simulink model "SOAR_integration_test"  (R2018b)
settings: Solver=VariableStepAuto  StartTime=0.0  StopTime=10.0  RelTol=1e-3
undefined symbols (not defined in the file): FSW_Lib, fswParams
libraries: sharedutil x3, dspmtrx3 x2, MEKF_lib x2, aerolibutil x2, actuators_lib x1, CDH_command_lib x1, Environment_lib x1, Mekf_joseph x1, actuator_processing_lib x1, allocation_lib x1, control_command_generation_lib x1, evironmentEstimation_lib x1
(part 1 of 2)
settings Model: Creator=devantormey  LastModifiedBy=devantormey

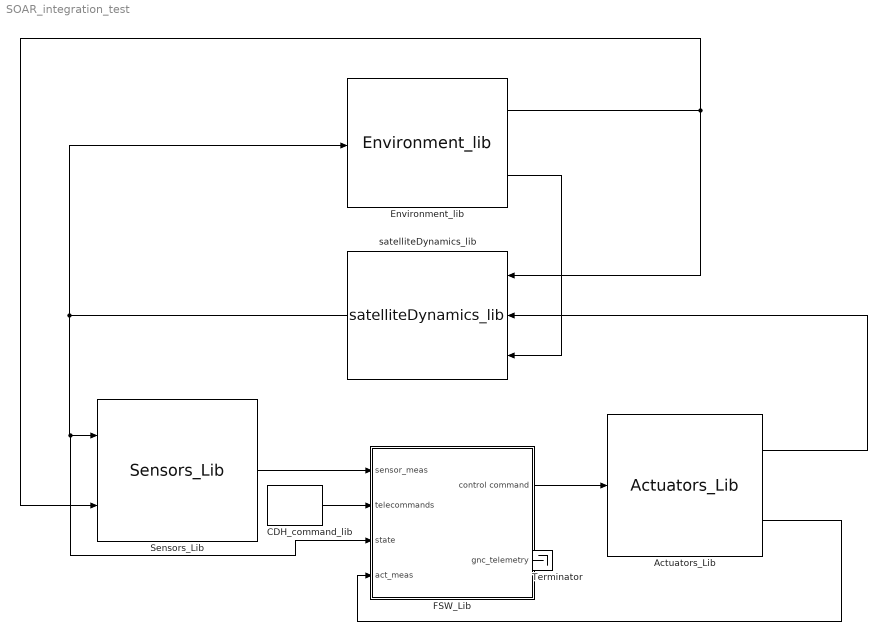
== system SOAR_integration_test ==
  Actuators_Lib : actuators_lib/Actuators_Lib  SystemSampleTime=-1
  CDH_command_lib : CDH_command_lib/CDH_command_lib  SystemSampleTime=-1
  Environment_lib : Environment_lib/Environment_lib  SystemSampleTime=-1
  FSW_Lib : Subsystem  AncestorBlock=FSW_Lib/FSW_Lib
  Sensors_Lib : Sensors_Lib/Sensors_Lib  SystemSampleTime=-1
  Terminator : Terminator
  satelliteDynamics_lib : satelliteDynamics_lib/satelliteDynamics_lib  SystemSampleTime=-1
  wires:
  Actuators_Lib/1 -> satelliteDynamics_lib/2
  FSW_Lib/2(gnc_telemetry) -> Terminator/1
  FSW_Lib/1(control command) -> Actuators_Lib/1
  Environment_lib/1 -> Sensors_Lib/2, satelliteDynamics_lib/1
  Environment_lib/2 -> satelliteDynamics_lib/3
  Sensors_Lib/1 -> FSW_Lib/1(sensor_meas)
  satelliteDynamics_lib/1 -> Environment_lib/1, FSW_Lib/3(state), Sensors_Lib/1
  Actuators_Lib/2 -> FSW_Lib/4(act_meas)
  CDH_command_lib/1 -> FSW_Lib/2(telecommands)

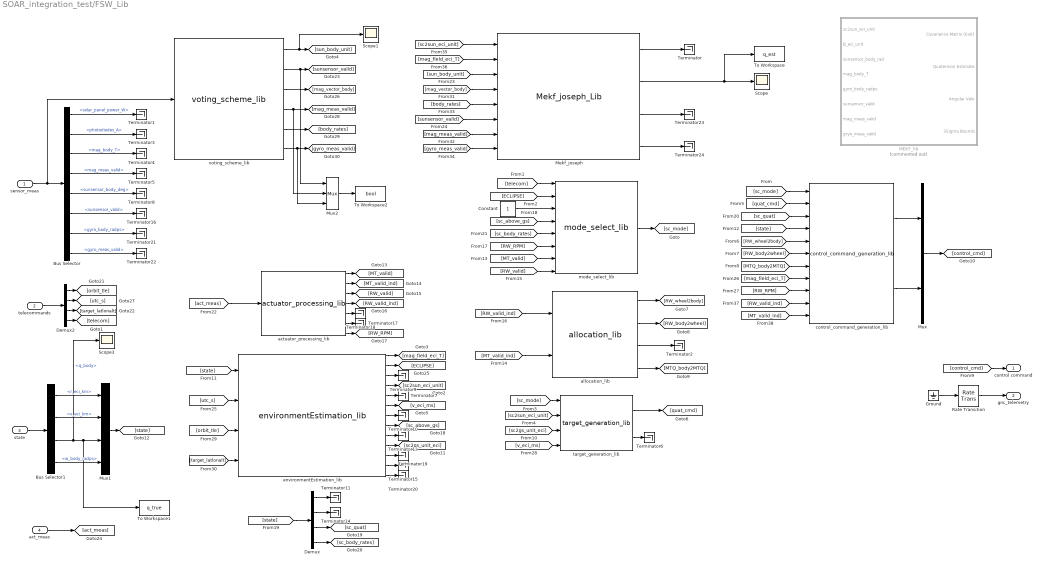
== system SOAR_integration_test/FSW_Lib ==
  sensor_meas : Inport
  telecommands : Inport  Port=2
  state : Inport  Port=3
  act_meas : Inport  Port=4
  Bus Selector : BusSelector  OutputSignals=solar_panel_power_W,photodiodes_A,mag_body_T,mag_meas_valid,sunsensor_body_deg,sunsensor_valid,gyro_body_radps,gyro_meas_valid
  Bus Selector1 : BusSelector  OutputSignals=r_eci_km,v_eci_km,q_body,w_body_radps
  Constant : Constant
  Demux : Demux  Outputs=[3 3 4 3]
  Demux2 : Demux  Outputs=[9 1 3 7]
  Ground : Ground
  MEKF_lib : Subsystem  Commented=on  AncestorBlock=MEKF_lib/MEKF_lib
  Mekf_joseph : Mekf_joseph/Mekf_joseph_Lib  SystemSampleTime=-1
      link override Data Store Memory: InitialValue=fswParams.estimation.ic.w_init
      link override "Subsystem Activated if: [Sun//Mag Sensor Invalid and Gyros are Valid] or [Gyro Invalid and Sun//Mag sensors Invalid]/TIME PROPAGATION of Q_EST, COVARIANCE": SourceBlock=Mekf_joseph/Mekf_joseph_Lib/Subsystem Activated if: [All Sensors Valid] or [Gyro Bad and Sun//Mag sensors Valid]/TIME PROPAGATION of Q_EST, COVARIANCE
  Mux : Mux  Inputs=[4 5]
  Mux1 : Mux  Inputs=[3;3;4;3]
  Mux2 : Mux  Inputs=3
  Rate Transition : RateTransition  OutPortSampleTime=fswParams.sample_time_s
  Scope : Scope
  Scope1 : Scope
  Scope3 : Scope
  Terminator{,1..11,13..24} (24 alike) : Terminator
  To Workspace : ToWorkspace  VariableName=q_est  SaveFormat=Timeseries  SampleTime=-1
  To Workspace1 : ToWorkspace  VariableName=q_true  SaveFormat=Timeseries  SampleTime=-1
  To Workspace2 : ToWorkspace  VariableName=bool  SaveFormat=Timeseries  SampleTime=-1
  actuator_processing_lib : actuator_processing_lib/actuator_processing_lib  SystemSampleTime=-1
  allocation_lib : allocation_lib/allocation_lib  SystemSampleTime=-1
  control_command_generation_lib : control_command_generation_lib/control_command_generation_lib  SystemSampleTime=-1
  environmentEstimation_lib : evironmentEstimation_lib/environmentEstimation_lib  SystemSampleTime=-1
      link override sgp4_lib_fsw/Gain: Gain=fswParams.constants.convert.KM2M
      link override sgp4_lib_fsw/Gain1: Gain=fswParams.constants.convert.KM2M
  mode_select_lib : mode_select_lib/mode_select_lib  SystemSampleTime=-1
  target_generation_lib : target_gen_lib/target_generation_lib  SystemSampleTime=-1
  voting_scheme_lib : voting_scheme_lib/voting_scheme_lib  SystemSampleTime=-1
  control command : Outport
  gnc_telemetry : Outport  Port=2
  wires:
  Rate Transition/1 -> gnc_telemetry/1
  target_generation_lib/1 -> [quat_cmd]
  [target_latlonalt] -> environmentEstimation_lib/4
  Demux2/3 -> [target_latlonalt]
  Demux2/1 -> [orbit_tle]
  [v_eci_ms] -> target_generation_lib/4
  [RW_RPM] -> control_command_generation_lib/9
  [mag_field_eci_T] -> control_command_generation_lib/8
  Demux2/2 -> [utc_s]
  Demux2/4 -> [telecom]
  environmentEstimation_lib/11 -> Terminator19/1
  environmentEstimation_lib/13 -> Terminator20/1
  environmentEstimation_lib/12 -> Terminator15/1
  Demux/2 -> Terminator14/1
  Demux/1 -> Terminator11/1
  Demux/4 -> [sc_body_rates]
  Demux/3 -> [sc_quat]
  [state] -> Demux/1
  actuator_processing_lib/7 -> [RW_RPM]
  actuator_processing_lib/6 -> Terminator17/1
  actuator_processing_lib/5 -> Terminator18/1
  actuator_processing_lib/4 -> [RW_valid_ind]
  actuator_processing_lib/3 -> [RW_valid]
  actuator_processing_lib/2 -> [MT_valid_ind]
  actuator_processing_lib/1 -> [MT_valid]
  act_meas/1 -> [act_meas]
  [state] -> control_command_generation_lib/4
  [state] -> environmentEstimation_lib/1
  [sc2gs_unit_eci] -> target_generation_lib/3
  [orbit_tle] -> environmentEstimation_lib/3
  [utc_s] -> environmentEstimation_lib/2
  environmentEstimation_lib/10 -> [sc2gs_unit_eci]
  environmentEstimation_lib/9 -> Terminator13/1
  environmentEstimation_lib/8 -> [sc_above_gs]
  environmentEstimation_lib/7 -> Terminator10/1
  environmentEstimation_lib/6 -> [v_eci_ms]
  environmentEstimation_lib/5 -> Terminator7/1
  environmentEstimation_lib/4 -> [sc2sun_eci_unit]
  environmentEstimation_lib/3 -> Terminator9/1
  environmentEstimation_lib/2 -> [ECLIPSE]
  environmentEstimation_lib/1 -> [mag_field_eci_T]
  Mux/1 -> [control_cmd]
  control_command_generation_lib/1 -> Mux/1
  control_command_generation_lib/2 -> Mux/2
  [MTQ_body2MTQ] -> control_command_generation_lib/7
  [RW_body2wheel] -> control_command_generation_lib/6
  allocation_lib/4 -> [MTQ_body2MTQ]
  allocation_lib/3 -> Terminator2/1
  [RW_wheel2body] -> control_command_generation_lib/5
  allocation_lib/2 -> [RW_body2wheel]
  allocation_lib/1 -> [RW_wheel2body]
  [sc_quat] -> control_command_generation_lib/3
  [MT_valid_ind] -> allocation_lib/2
  [RW_valid_ind] -> allocation_lib/1
  [quat_cmd] -> control_command_generation_lib/2
  target_generation_lib/2 -> Terminator6/1
  [sc2sun_eci_unit] -> target_generation_lib/2
  [sc_mode] -> target_generation_lib/1
  [RW_valid] -> mode_select_lib/8
  [MT_valid] -> mode_select_lib/7
  Constant/1 -> mode_select_lib/3
  [RW_RPM] -> mode_select_lib/6
  [sc_body_rates] -> mode_select_lib/5
  [sc_above_gs] -> mode_select_lib/4
  [ECLIPSE] -> mode_select_lib/2
  [telecom] -> mode_select_lib/1
  [sc_mode] -> control_command_generation_lib/1
  mode_select_lib/1 -> [sc_mode]
  [control_cmd] -> control command/1
  Ground/1 -> Rate Transition/1
  telecommands/1 -> Demux2/1
  sensor_meas/1 -> voting_scheme_lib/1, Bus Selector/1
  Bus Selector/1 -> Terminator1/1  "<solar_panel_power_W>"
  Bus Selector/2 -> Terminator3/1  "<photodiodes_A>"
  Bus Selector/3 -> Terminator4/1  "<mag_body_T>"
  Bus Selector/4 -> Terminator5/1  "<mag_meas_valid>"
  Bus Selector/5 -> Terminator8/1  "<sunsensor_body_deg>"
  Bus Selector/6 -> Terminator16/1  "<sunsensor_valid>"
  Bus Selector/7 -> Terminator21/1  "<gyro_body_radps>"
  Bus Selector/8 -> Terminator22/1  "<gyro_meas_valid>"
  voting_scheme_lib/3 -> [mag_vector_body]
  voting_scheme_lib/4 -> Mux2/2, [mag_meas_valid]
  voting_scheme_lib/5 -> [body_rates]
  voting_scheme_lib/6 -> Mux2/3, [gyro_meas_valid]
  [act_meas] -> actuator_processing_lib/1
  voting_scheme_lib/1 -> Scope1/1, [sun_body_unit]
  state/1 -> Bus Selector1/1
  Bus Selector1/1 -> Mux1/1  "<r_eci_km>"
  Bus Selector1/2 -> Mux1/2  "<v_eci_km>"
  Bus Selector1/3 -> To Workspace1/1, Mux1/3, Scope3/1  "<q_body>"
  Bus Selector1/4 -> Mux1/4  "<w_body_radps>"
  Mux1/1 -> [state]
  [sc2sun_eci_unit] -> Mekf_joseph/1
  [mag_field_eci_T] -> Mekf_joseph/2
  [body_rates] -> Mekf_joseph/5
  [mag_vector_body] -> Mekf_joseph/4
  [sunsensor_valid] -> Mekf_joseph/6
  [mag_meas_valid] -> Mekf_joseph/7
  [gyro_meas_valid] -> Mekf_joseph/8
  [sun_body_unit] -> Mekf_joseph/3
  Mekf_joseph/1 -> Terminator/1
  Mekf_joseph/2 -> Scope/1, To Workspace/1
  Mekf_joseph/3 -> Terminator23/1
  Mekf_joseph/4 -> Terminator24/1
  Mux2/1 -> To Workspace2/1
  voting_scheme_lib/2 -> Mux2/1, [sunsensor_valid]
  [RW_valid_ind] -> control_command_generation_lib/10
  [MT_valid_ind] -> control_command_generation_lib/11

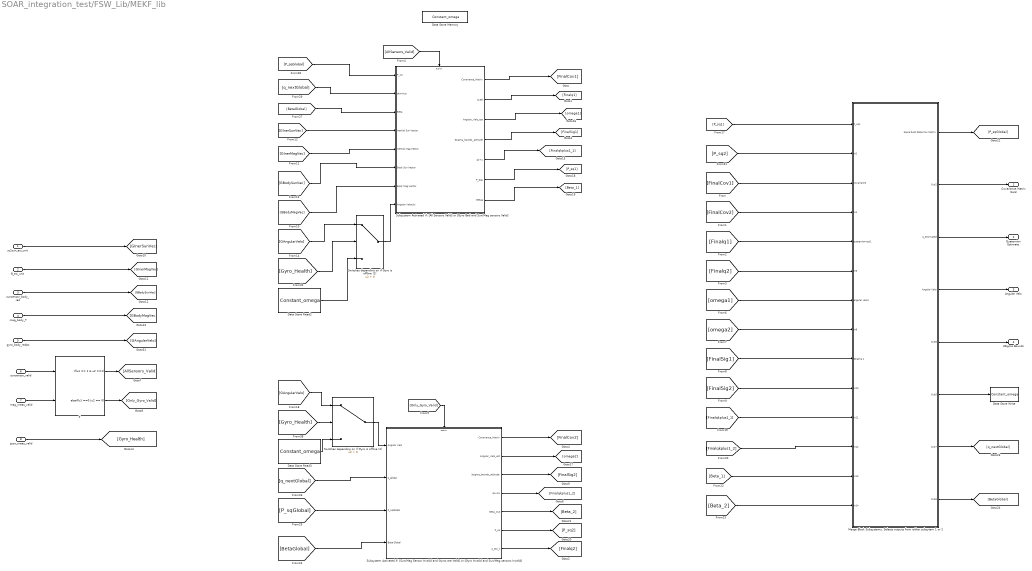
== system SOAR_integration_test/FSW_Lib/MEKF_lib ==
  sc2sun_eci_unit : Inport
  B_eci_unit : Inport  Port=2
  sunsensor_body_rad : Inport  Port=3
  mag_body_T : Inport  Port=4
  gyro_body_radps : Inport  Port=5
  sunsensor_valid : Inport  Port=6
  mag_meas_valid : Inport  Port=7
  gryo_meas_valid : Inport  Port=8
  Data Store Memory : DataStoreMemory  DataStoreName=Constant_omega  ReadBeforeWriteMsg=warning  WriteAfterWriteMsg=warning  WriteAfterReadMsg=warning  InitialValue=fswParams.estimation.ic.w_init  VectorParams1D=off  ShowAdditionalParam=off
  Data Store Read2 : DataStoreRead  DataStoreName=Constant_omega
  Data Store Read3 : DataStoreRead  DataStoreName=Constant_omega
  Data Store Write : DataStoreWrite  DataStoreName=Constant_omega
  If : If  NumInputs=2  IfExpression=u1 == 1 & u2 ==1  ElseIfExpressions=u1 ==0 |u2 == 0  ShowElse=off
  "Merge Block Subsystems, Selects outputs from either subsytem 1 or 2" : Subsystem
  Subsystem Activated if: [All Sensors Valid] or [Gyro Bad and Sun/Mag sensors Valid] : Subsystem  TreatAsAtomicUnit=on
  Subsystem Activated if: [Sun/Mag Sensor Invalid and Gyros are Valid] or [Gyro Invalid and Sun/Mag sensors Invalid] : Subsystem  TreatAsAtomicUnit=on
  Switches depending on if Gyro is offline (1) : Switch  Criteria=u2 > Threshold
  Switches depending on if Gyro is offline (2) : Switch  Criteria=u2 > Threshold
  Covariance Matrix (6x6) : Outport
  "Quaternion Estimate " : Outport  Port=2
  "Angular Velo " : Outport  Port=3
  "3Sigma Bounds " : Outport  Port=4
  wires:
  gyro_body_radps/1 -> [GAngularVelo]
  mag_body_T/1 -> [GBodyMagVec]
  B_eci_unit/1 -> [GInerMagVec]
  gryo_meas_valid/1 -> [Gyro_Health]
  mag_meas_valid/1 -> If/2
  sunsensor_valid/1 -> If/1
  sunsensor_body_rad/1 -> [GBodySunVec]
  sc2sun_eci_unit/1 -> [GInerSunVec]
  "Merge Block Subsystems, Selects outputs from either subsytem 1 or 2"/8(Out8) -> [BetaGlobal]
  "Merge Block Subsystems, Selects outputs from either subsytem 1 or 2"/7(Out7) -> [q_nextGlobal]
  "Merge Block Subsystems, Selects outputs from either subsytem 1 or 2"/5(Out6) -> "3Sigma Bounds "/1
  "Merge Block Subsystems, Selects outputs from either subsytem 1 or 2"/6(Out5) -> Data Store Write/1
  "Merge Block Subsystems, Selects outputs from either subsytem 1 or 2"/4(Angular Velo) -> "Angular Velo "/1
  "Merge Block Subsystems, Selects outputs from either subsytem 1 or 2"/3(q_estimated) -> "Quaternion Estimate "/1
  "Merge Block Subsystems, Selects outputs from either subsytem 1 or 2"/2(Out2) -> Covariance Matrix (6x6)/1
  "Merge Block Subsystems, Selects outputs from either subsytem 1 or 2"/1(Squre Root State Cov Matrix) -> [P_sqGlobal]
  [Beta_2] -> "Merge Block Subsystems, Selects outputs from either subsytem 1 or 2"/14(In14)
  [Beta_1] -> "Merge Block Subsystems, Selects outputs from either subsytem 1 or 2"/13(In13)
  [Finalqkplus1_2] -> "Merge Block Subsystems, Selects outputs from either subsytem 1 or 2"/12(In12)
  [Finalqkplus1_1] -> "Merge Block Subsystems, Selects outputs from either subsytem 1 or 2"/11(In11)
  [FinalSig2] -> "Merge Block Subsystems, Selects outputs from either subsytem 1 or 2"/10(In10)
  [FinalSig1] -> "Merge Block Subsystems, Selects outputs from either subsytem 1 or 2"/9(3sigma 1)
  [omega2] -> "Merge Block Subsystems, Selects outputs from either subsytem 1 or 2"/8(In8)
  [omega1] -> "Merge Block Subsystems, Selects outputs from either subsytem 1 or 2"/7(angular velo1)
  [Finalq2] -> "Merge Block Subsystems, Selects outputs from either subsytem 1 or 2"/6(In6)
  [Finalq1] -> "Merge Block Subsystems, Selects outputs from either subsytem 1 or 2"/5(quaternion est1)
  [FinalCov2] -> "Merge Block Subsystems, Selects outputs from either subsytem 1 or 2"/4(In4)
  [FinalCov1] -> "Merge Block Subsystems, Selects outputs from either subsytem 1 or 2"/3(covariance)
  [P_sq2] -> "Merge Block Subsystems, Selects outputs from either subsytem 1 or 2"/2(In2)
  [P_sq1] -> "Merge Block Subsystems, Selects outputs from either subsytem 1 or 2"/1(P_sq1)
  Switches depending on if Gyro is offline (2)/1 -> Subsystem Activated if: [Sun/Mag Sensor Invalid and Gyros are Valid] or [Gyro Invalid and Sun/Mag sensors Invalid]/1(Angular Velo)
  Data Store Read3/1 -> Switches depending on if Gyro is offline (2)/3
  [GAngularVelo] -> Switches depending on if Gyro is offline (2)/1
  [Gyro_Health] -> Switches depending on if Gyro is offline (2)/2
  Switches depending on if Gyro is offline (1)/1 -> Subsystem Activated if: [All Sensors Valid] or [Gyro Bad and Sun/Mag sensors Valid]/8(Angular Velocity)
  Data Store Read2/1 -> Switches depending on if Gyro is offline (1)/3
  [Gyro_Health] -> Switches depending on if Gyro is offline (1)/2
  [GAngularVelo] -> Switches depending on if Gyro is offline (1)/1
  If/2 -> [Only_Gyro_Valid]
  If/1 -> [AllSensors_Valid]
  [P_sqGlobal] -> Subsystem Activated if: [All Sensors Valid] or [Gyro Bad and Sun/Mag sensors Valid]/1(P_sq)
  [q_nextGlobal] -> Subsystem Activated if: [All Sensors Valid] or [Gyro Bad and Sun/Mag sensors Valid]/2(qkminus)
  Subsystem Activated if: [Sun/Mag Sensor Invalid and Gyros are Valid] or [Gyro Invalid and Sun/Mag sensors Invalid]/2(Angular_Velo_est) -> [omega2]
  Subsystem Activated if: [Sun/Mag Sensor Invalid and Gyros are Valid] or [Gyro Invalid and Sun/Mag sensors Invalid]/5(Beta_Out) -> [Beta_2]
  Subsystem Activated if: [Sun/Mag Sensor Invalid and Gyros are Valid] or [Gyro Invalid and Sun/Mag sensors Invalid]/6(P_sq) -> [P_sq2]
  Subsystem Activated if: [All Sensors Valid] or [Gyro Bad and Sun/Mag sensors Valid]/7(Betaa) -> [Beta_1]
  Subsystem Activated if: [All Sensors Valid] or [Gyro Bad and Sun/Mag sensors Valid]/6("P_Sqa ") -> [P_sq1]
  Subsystem Activated if: [All Sensors Valid] or [Gyro Bad and Sun/Mag sensors Valid]/3(Angular_Velo_est) -> [omega1]
  [BetaGlobal] -> Subsystem Activated if: [All Sensors Valid] or [Gyro Bad and Sun/Mag sensors Valid]/3(Beta)
  [BetaGlobal] -> Subsystem Activated if: [Sun/Mag Sensor Invalid and Gyros are Valid] or [Gyro Invalid and Sun/Mag sensors Invalid]/4(Beta Global)
  [P_sqGlobal] -> Subsystem Activated if: [Sun/Mag Sensor Invalid and Gyros are Valid] or [Gyro Invalid and Sun/Mag sensors Invalid]/3(P_sqGlobal)
  Subsystem Activated if: [All Sensors Valid] or [Gyro Bad and Sun/Mag sensors Valid]/5(qk+1) -> [Finalqkplus1_1]
  [q_nextGlobal] -> Subsystem Activated if: [Sun/Mag Sensor Invalid and Gyros are Valid] or [Gyro Invalid and Sun/Mag sensors Invalid]/2(q_global)
  Subsystem Activated if: [Sun/Mag Sensor Invalid and Gyros are Valid] or [Gyro Invalid and Sun/Mag sensors Invalid]/3(3sigma_bounds_attitude) -> [FinalSig2]
  [AllSensors_Valid] -> Subsystem Activated if: [All Sensors Valid] or [Gyro Bad and Sun/Mag sensors Valid]/Action
  Subsystem Activated if: [Sun/Mag Sensor Invalid and Gyros are Valid] or [Gyro Invalid and Sun/Mag sensors Invalid]/1(Covariance_Matrix) -> [FinalCov2]
  [GInerSunVec] -> Subsystem Activated if: [All Sensors Valid] or [Gyro Bad and Sun/Mag sensors Valid]/4(Inertial Sun Vector)
  Subsystem Activated if: [Sun/Mag Sensor Invalid and Gyros are Valid] or [Gyro Invalid and Sun/Mag sensors Invalid]/7(q_est_k) -> [Finalq2]
  Subsystem Activated if: [All Sensors Valid] or [Gyro Bad and Sun/Mag sensors Valid]/4(3sigma_bounds_attitude) -> [FinalSig1]
  [Only_Gyro_Valid] -> Subsystem Activated if: [Sun/Mag Sensor Invalid and Gyros are Valid] or [Gyro Invalid and Sun/Mag sensors Invalid]/Action
  Subsystem Activated if: [All Sensors Valid] or [Gyro Bad and Sun/Mag sensors Valid]/1(Covariance_Matrix) -> [FinalCov1]
  Subsystem Activated if: [All Sensors Valid] or [Gyro Bad and Sun/Mag sensors Valid]/2(q_est) -> [Finalq1]
  Subsystem Activated if: [Sun/Mag Sensor Invalid and Gyros are Valid] or [Gyro Invalid and Sun/Mag sensors Invalid]/4(qk+1a) -> [Finalqkplus1_2]
  [GBodyMagVec] -> Subsystem Activated if: [All Sensors Valid] or [Gyro Bad and Sun/Mag sensors Valid]/7(Body Mag Vector)
  [GInerMagVec] -> Subsystem Activated if: [All Sensors Valid] or [Gyro Bad and Sun/Mag sensors Valid]/5(Inertial Mag Vector)
  [GBodySunVec] -> Subsystem Activated if: [All Sensors Valid] or [Gyro Bad and Sun/Mag sensors Valid]/6(Body Sun Vector)

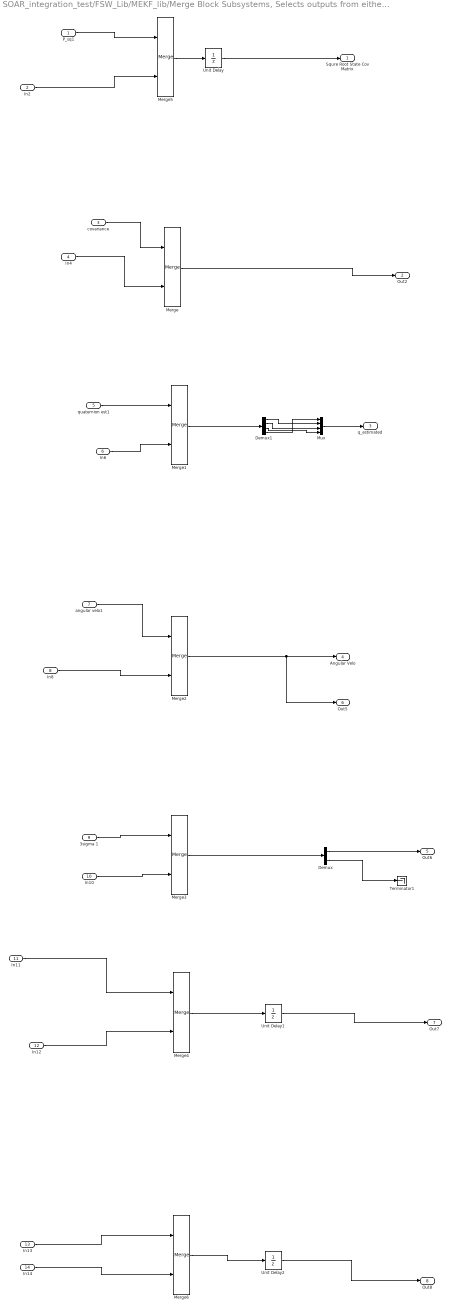
== system SOAR_integration_test/FSW_Lib/MEKF_lib/Merge Block Subsystems, Selects outputs from either subsytem 1 or 2 ==
  P_sq1 : Inport
  In2 : Inport  Port=2
  covariance : Inport  Port=3
  In4 : Inport  Port=4
  quaternion est1 : Inport  Port=5
  In6 : Inport  Port=6
  angular velo1 : Inport  Port=7
  In8 : Inport  Port=8
  3sigma 1 : Inport  Port=9
  In10 : Inport  Port=10
  In11 : Inport  Port=11
  In12 : Inport  Port=12
  In13 : Inport  Port=13
  In14 : Inport  Port=14
  Demux : Demux  Outputs=2
  Demux1 : Demux
  Merge{,1..6} (7 alike) : Merge
  Mux : Mux
  Terminator1 : Terminator
  Unit Delay : UnitDelay  InitialCondition=fswParams.estimation.ic.P_sq_init  SampleTime=-1
  Unit Delay1 : UnitDelay  InitialCondition=fswParams.estimation.ic.quat_est_init  SampleTime=-1
  Unit Delay2 : UnitDelay  InitialCondition=fswParams.estimation.ic.Beta_init  SampleTime=-1
  Squre Root State Cov Matrix : Outport
  Out2 : Outport  Port=2
  q_estimated : Outport  Port=3
  Angular Velo : Outport  Port=4
  Out6 : Outport  Port=5
  Out5 : Outport  Port=6
  Out7 : Outport  Port=7
  Out8 : Outport  Port=8
  wires:
  Mux/1 -> q_estimated/1
  Demux1/3 -> Mux/4
  Demux1/2 -> Mux/3
  Demux1/1 -> Mux/2
  Demux1/4 -> Mux/1
  Merge1/1 -> Demux1/1
  Unit Delay/1 -> Squre Root State Cov Matrix/1
  Unit Delay2/1 -> Out8/1
  P_sq1/1 -> Merge5/1
  In12/1 -> Merge4/2
  In8/1 -> Merge2/2
  In6/1 -> Merge1/2
  Merge/1 -> Out2/1
  In13/1 -> Merge6/1
  Demux/1 -> Out6/1
  In4/1 -> Merge/2
  Merge4/1 -> Unit Delay1/1
  covariance/1 -> Merge/1
  In2/1 -> Merge5/2
  In10/1 -> Merge3/2
  Merge5/1 -> Unit Delay/1
  In11/1 -> Merge4/1
  angular velo1/1 -> Merge2/1
  In14/1 -> Merge6/2
  quaternion est1/1 -> Merge1/1
  3sigma 1/1 -> Merge3/1
  Merge6/1 -> Unit Delay2/1
  Demux/2 -> Terminator1/1
  Unit Delay1/1 -> Out7/1
  Merge2/1 -> Angular Velo/1, Out5/1
  Merge3/1 -> Demux/1

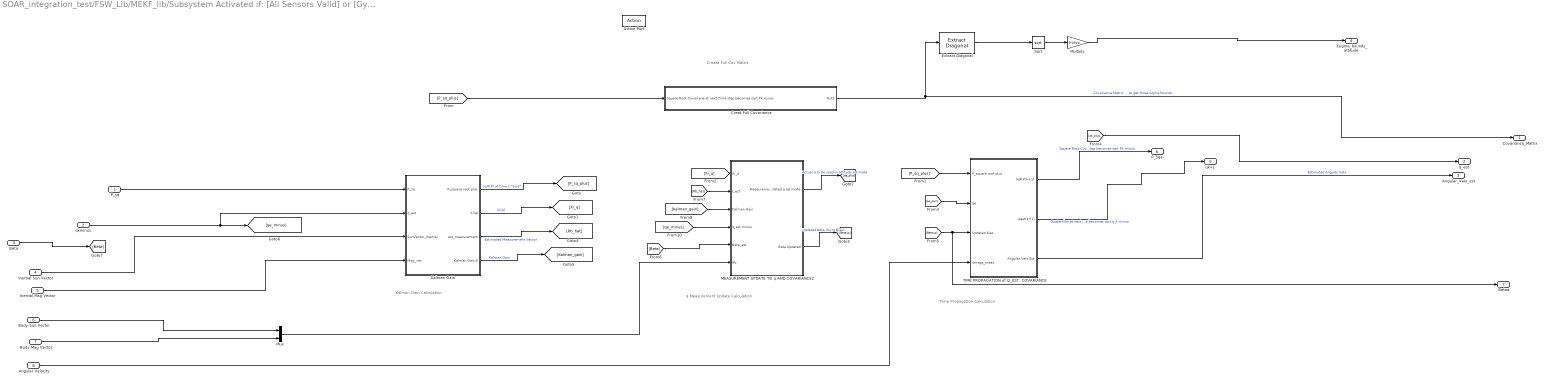
== system SOAR_integration_test/FSW_Lib/MEKF_lib/Subsystem Activated if: [All Sensors Valid] or [Gyro Bad and Sun//Mag sensors Valid] ==
  note: q Measurement Update Calculation
  note: Create Full Cov Matrix
  note: Time Propagation Calculation
  note: Kalman Gain Calculation
  P_sq : Inport
  qkminus : Inport  Port=2
  Beta : Inport  Port=3
  Inertial Sun Vector : Inport  Port=4
  Inertial Mag Vector : Inport  Port=5
  Body Sun Vector : Inport  Port=6
  Body Mag Vector : Inport  Port=7
  Angular Velocity : Inport  Port=8
  Action Port : ActionPort
  Creat Full Covariance : Subsystem  AncestorBlock=MEKF_LibraryR2018b/Multiplicative Extended Kalman Filter/Creat Full Covariance
  Extract Diagonal : dspmtrx3/Extract Diagonal
      settings: SourceProductName=DSP System Toolbox  SourceProductBaseCode=DS
  Kalman Gain : Subsystem  AncestorBlock=MEKF_LibraryR2018b/Multiplicative Extended Kalman Filter/Kalman Gain
  MEASUREMENT UPDATE TO q AND COVARIANCE2 : Subsystem  AncestorBlock=MEKF_LibraryR2018b/Multiplicative Extended Kalman Filter/MEASUREMENT UPDATE TO q AND COVARIANCE2
  Multiply : Gain  Gain=3*180/pi
  Mux : Mux  Inputs=2
  Sqrt : Sqrt  SaturateOnIntegerOverflow=on
  "TIME PROPAGATION of Q_EST, COVARIANCE" : Subsystem  AncestorBlock=MEKF_Library/Multiplicative Extended Kalman Filter/TIME PROPAGATION of Q_EST, COVARIANCE
  Covariance_Matrix : Outport
  q_est : Outport  Port=2
  Angular_Velo_est : Outport  Port=3
  3sigma_bounds_attitude : Outport  Port=4
  qk+1 : Outport  Port=5
  "P_Sqa " : Outport  Port=6
  Betaa : Outport  Port=7
  wires:
  Beta/1 -> [Beta]
  Multiply/1 -> 3sigma_bounds_attitude/1
  Mux/1 -> MEASUREMENT UPDATE TO q AND COVARIANCE2/6(Rb)
  Body Mag Vector/1 -> Mux/2
  Body Sun Vector/1 -> Mux/1
  Inertial Mag Vector/1 -> Kalman Gain/4("Mag_vec ")
  [Kalman_gain] -> MEASUREMENT UPDATE TO q AND COVARIANCE2/3(Kalman Gain)
  [Xi_q] -> MEASUREMENT UPDATE TO q AND COVARIANCE2/1(Xi_q)
  Kalman Gain/3(est_measurement) -> [Rb_hat]  "Estimated Measurement Vector"
  [P_sq_plus] -> "TIME PROPAGATION of Q_EST, COVARIANCE"/1(P_square root plus)
  MEASUREMENT UPDATE TO q AND COVARIANCE2/1(Measurement updated q estimate) -> [qe_plus]  "Actual q to be used in attitude estimate"
  [Beta] -> MEASUREMENT UPDATE TO q AND COVARIANCE2/5(Beta_est)
  [Betaup] -> "TIME PROPAGATION of Q_EST, COVARIANCE"/3(Updated bias), Betaa/1
  [P_sq_plus] -> Creat Full Covariance/1(Square Root Covariane at next Time step becomes sqrt Pk minus)
  Sqrt/1 -> Multiply/1
  Kalman Gain/2(Xi(q)) -> [Xi_q]  "Xi(q)"
  [qe_minus] -> MEASUREMENT UPDATE TO q AND COVARIANCE2/4(q_est minus)
  Kalman Gain/4(Kalman Gain K) -> [Kalman_gain]  "Kalman Gain"
  Kalman Gain/1(P_square root plus) -> [P_sq_plus]  "sqrt(P) at time k *plus*"
  "TIME PROPAGATION of Q_EST, COVARIANCE"/1(SqR P(k+1)) -> "P_Sqa "/1  "Square Root Covariane at next Time step becomes sqrt Pk minus"
  [Rb_hat] -> MEASUREMENT UPDATE TO q AND COVARIANCE2/2(r_est)
  MEASUREMENT UPDATE TO q AND COVARIANCE2/2(Beta Updated) -> [Betaup]  "Updated Beta (Gyro Bias)"
  [qe_plus] -> "TIME PROPAGATION of Q_EST, COVARIANCE"/2(qe)
  P_sq/1 -> Kalman Gain/1(P_sq)
  Angular Velocity/1 -> "TIME PROPAGATION of Q_EST, COVARIANCE"/4(omega_meas)
  Extract Diagonal/1 -> Sqrt/1
  qkminus/1 -> [qe_minus], Kalman Gain/2(q_est)
  Creat Full Covariance/1(Out1) -> Extract Diagonal/1, Covariance_Matrix/1  "Covariance Matrix from which to get three sigma bounds"
  "TIME PROPAGATION of Q_EST, COVARIANCE"/3(Angular Velo Est) -> Angular_Velo_est/1  "Estimated Angular Velo"
  "TIME PROPAGATION of Q_EST, COVARIANCE"/2(qest(k+1)) -> qk+1/1  "Quaternion at next Time step becomes sqrt q_k minus"
  [qe_plus] -> q_est/1
  Inertial Sun Vector/1 -> Kalman Gain/3(SunVector_Inertial)

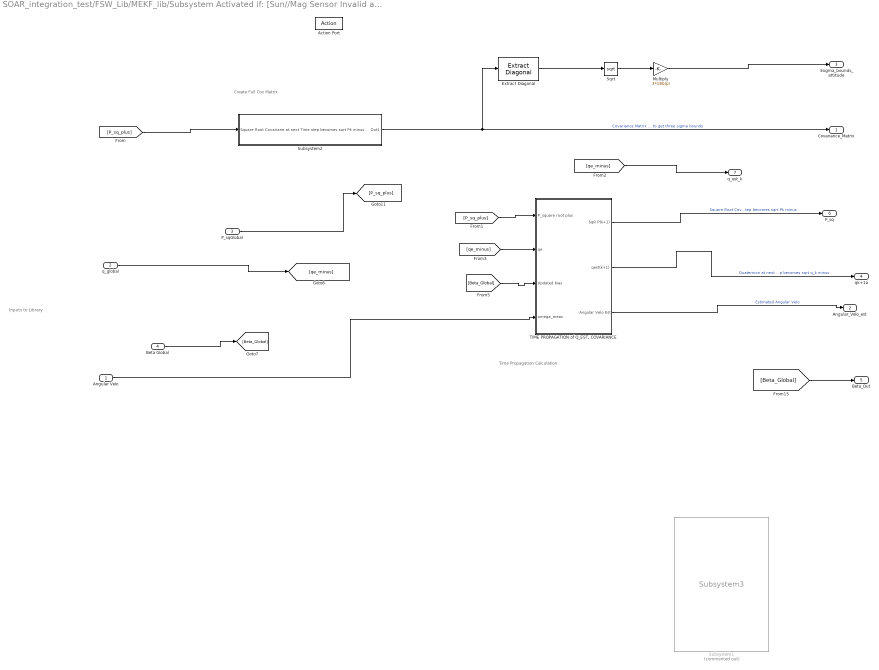
== system SOAR_integration_test/FSW_Lib/MEKF_lib/Subsystem Activated if: [Sun//Mag Sensor Invalid and Gyros are Valid] or [Gyro Invalid and Sun//Mag sensors Invalid] ==
  note: Time Propagation Calculation
  note: Inputs to Library
  note: Create Full Cov Matrix
  Angular Velo : Inport
  q_global : Inport  Port=2
  P_sqGlobal : Inport  Port=3
  Beta Global : Inport  Port=4
  Action Port : ActionPort
  Extract Diagonal : dspmtrx3/Extract Diagonal
      settings: SourceProductName=DSP System Toolbox  SourceProductBaseCode=DS
  Multiply : Gain  Gain=3*180/pi
  Sqrt : Sqrt  SaturateOnIntegerOverflow=on
  Subsystem1 : MEKF_lib/MEKF with Validity Check/Subsystem Activated if: [Sun//Mag Sensor Invalid and Gyros are Valid] or [Gyro Invalid and Sun//Mag sensors Invalid]/Subsystem3  Commented=on  SystemSampleTime=-1  SSRTWFcnClass=[]
  Subsystem2 : Subsystem
  "TIME PROPAGATION of Q_EST, COVARIANCE" : Subsystem  AncestorBlock=|
      | MEKF_SensorCheck_Lib2018/MEKF with Validity Check/Subsystem Activated if: [All Sensors Valid]
      | or
      | [Gyro Bad and Sun//Mag sensors Valid]/TIME PROPAGATION of Q_EST, COVARIANCE
  Covariance_Matrix : Outport
  Angular_Velo_est : Outport  Port=2
  3sigma_bounds_attitude : Outport  Port=3
  qk+1a : Outport  Port=4
  Beta_Out : Outport  Port=5
  P_sq : Outport  Port=6
  q_est_k : Outport  Port=7
  wires:
  [qe_minus] -> q_est_k/1
  [Beta_Global] -> Beta_Out/1
  Beta Global/1 -> [Beta_Global]
  "TIME PROPAGATION of Q_EST, COVARIANCE"/1(SqR P(k+1)) -> P_sq/1  "Square Root Covariane at next Time step becomes sqrt Pk minus"
  Multiply/1 -> 3sigma_bounds_attitude/1
  Angular Velo/1 -> "TIME PROPAGATION of Q_EST, COVARIANCE"/4(omega_meas)
  q_global/1 -> [qe_minus]
  Extract Diagonal/1 -> Sqrt/1
  [Beta_Global] -> "TIME PROPAGATION of Q_EST, COVARIANCE"/3(Updated bias)
  [P_sq_plus] -> "TIME PROPAGATION of Q_EST, COVARIANCE"/1(P_square root plus)
  [P_sq_plus] -> Subsystem2/1(Square Root Covariane at next Time step becomes sqrt Pk minus)
  "TIME PROPAGATION of Q_EST, COVARIANCE"/3(Angular Velo Est) -> Angular_Velo_est/1  "Estimated Angular Velo"
  Subsystem2/1(Out1) -> Extract Diagonal/1, Covariance_Matrix/1  "Covariance Matrix from which to get three sigma bounds"
  Sqrt/1 -> Multiply/1
  "TIME PROPAGATION of Q_EST, COVARIANCE"/2(qest(k+1)) -> qk+1a/1  "Quaternion at next Time step becomes sqrt q_k minus"
  [qe_minus] -> "TIME PROPAGATION of Q_EST, COVARIANCE"/2(qe)
  P_sqGlobal/1 -> [P_sq_plus]

== system SOAR_integration_test/FSW_Lib/MEKF_lib/Subsystem Activated if: [All Sensors Valid] or [Gyro Bad and Sun//Mag sensors Valid]/Creat Full Covariance ==
  Square Root Covariane at next Time step becomes sqrt Pk minus : Inport
  Matrix Multiply : Product  Multiplication=Matrix(*)
  Transpose : Math  Operator=transpose  SaturateOnIntegerOverflow=on
  Out1 : Outport
  wires:
  Matrix Multiply/1 -> Out1/1
  Transpose/1 -> Matrix Multiply/2
  Square Root Covariane at next Time step becomes sqrt Pk minus/1 -> Matrix Multiply/1, Transpose/1

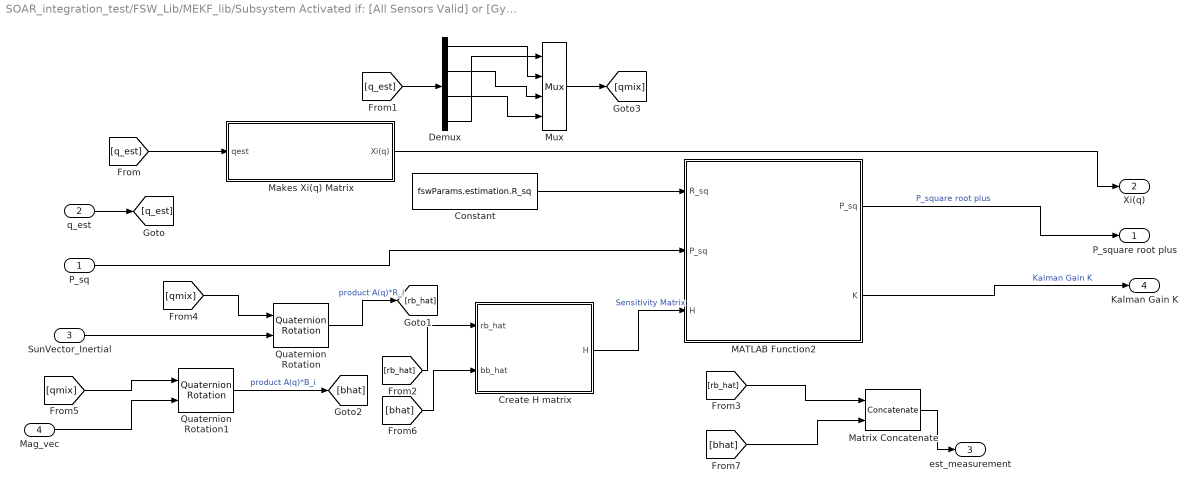
== system SOAR_integration_test/FSW_Lib/MEKF_lib/Subsystem Activated if: [All Sensors Valid] or [Gyro Bad and Sun//Mag sensors Valid]/Kalman Gain ==
  P_sq : Inport
  q_est : Inport  Port=2
  SunVector_Inertial : Inport  Port=3
  "Mag_vec " : Inport  Port=4
  Constant : Constant  Value=fswParams.estimation.R_sq  VectorParams1D=off
  Create H matrix : Subsystem
  Demux : Demux
  MATLAB Function2 : MATLAB Function  TreatAsAtomicUnit=on
  Makes Xi(q) Matrix : Subsystem
  Matrix Concatenate : Concatenate  Mode=Multidimensional array
  Mux : Mux
  Quaternion Rotation : aerolibutil/Quaternion Rotation
  Quaternion Rotation1 : aerolibutil/Quaternion Rotation
  P_square root plus : Outport
  Xi(q) : Outport  Port=2
  est_measurement : Outport  Port=3
  Kalman Gain K : Outport  Port=4
  wires:
  Matrix Concatenate/1 -> est_measurement/1
  [bhat] -> Matrix Concatenate/2
  [rb_hat] -> Matrix Concatenate/1
  [bhat] -> Create H matrix/2(bb_hat)
  [qmix] -> Quaternion Rotation/1
  [qmix] -> Quaternion Rotation1/1
  Mux/1 -> [qmix]
  Quaternion Rotation1/1 -> [bhat]  "product A(q)*B_i"
  "Mag_vec "/1 -> Quaternion Rotation1/2
  [rb_hat] -> Create H matrix/1(rb_hat)
  Quaternion Rotation/1 -> [rb_hat]  "product A(q)*R_i"
  [q_est] -> Makes Xi(q) Matrix/1(qest)
  [q_est] -> Demux/1
  q_est/1 -> [q_est]
  Makes Xi(q) Matrix/1(Xi(q)) -> Xi(q)/1
  Demux/4 -> Mux/1
  Demux/3 -> Mux/4
  Demux/2 -> Mux/3
  Demux/1 -> Mux/2
  MATLAB Function2/1(P_sq) -> P_square root plus/1  "P_square root plus"
  Constant/1 -> MATLAB Function2/1(R_sq)
  SunVector_Inertial/1 -> Quaternion Rotation/2
  MATLAB Function2/2(K) -> Kalman Gain K/1  "Kalman Gain K"
  P_sq/1 -> MATLAB Function2/2("P_sq ")
  Create H matrix/1(H) -> MATLAB Function2/3(H)  "Sensitivity Matrix"

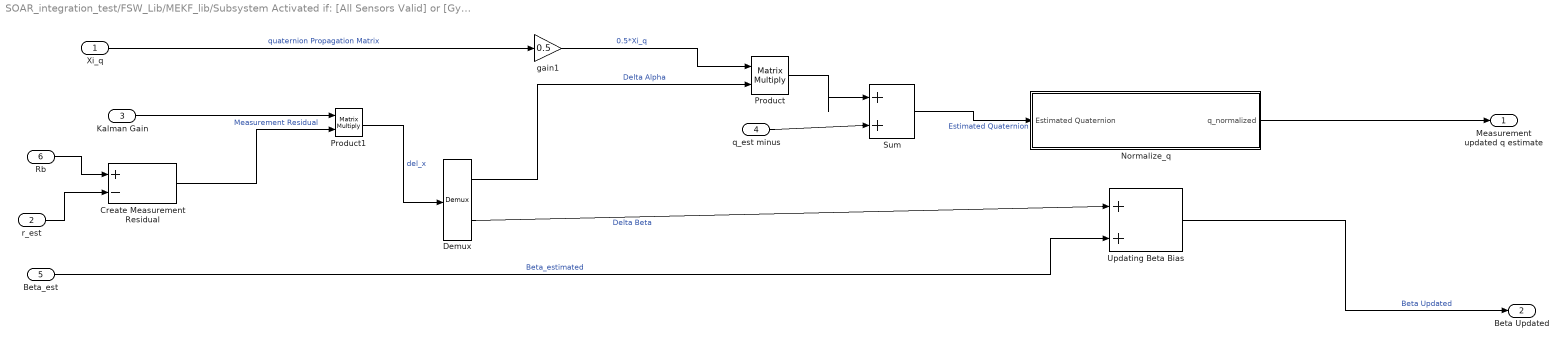
== system SOAR_integration_test/FSW_Lib/MEKF_lib/Subsystem Activated if: [All Sensors Valid] or [Gyro Bad and Sun//Mag sensors Valid]/MEASUREMENT UPDATE TO q AND COVARIANCE2 ==
  Xi_q : Inport
  r_est : Inport  Port=2
  Kalman Gain : Inport  Port=3
  q_est minus : Inport  Port=4
  Beta_est : Inport  Port=5
  Rb : Inport  Port=6
  Create Measurement Residual : Sum  Inputs=+-
  Demux : Demux  Outputs=2
  Normalize_q : Subsystem
  Product : Product  Inputs=**  Multiplication=Matrix(*)
  Product1 : Product  Multiplication=Matrix(*)
  Sum : Sum  Inputs=|++
  "Updating Beta Bias " : Sum  Inputs=|++
  gain1 : Gain  Gain=0.5
  Measurement updated q estimate : Outport
  Beta Updated : Outport  Port=2
  wires:
  Normalize_q/1(q_normalized) -> Measurement updated q estimate/1
  Sum/1 -> Normalize_q/1(Estimated Quaternion)  "Estimated Quaternion"
  Xi_q/1 -> gain1/1  "quaternion Propagation Matrix"
  Rb/1 -> Create Measurement Residual/1
  Kalman Gain/1 -> Product1/1
  q_est minus/1 -> Sum/2
  Beta_est/1 -> "Updating Beta Bias "/2  "Beta_estimated"
  "Updating Beta Bias "/1 -> Beta Updated/1  "Beta Updated"
  Create Measurement Residual/1 -> Product1/2  "Measurement Residual"
  r_est/1 -> Create Measurement Residual/2
  Product1/1 -> Demux/1  "del_x"
  Product/1 -> Sum/1
  Demux/2 -> "Updating Beta Bias "/1  "Delta Beta"
  gain1/1 -> Product/1  "0.5*Xi_q"
  Demux/1 -> Product/2  "Delta Alpha"

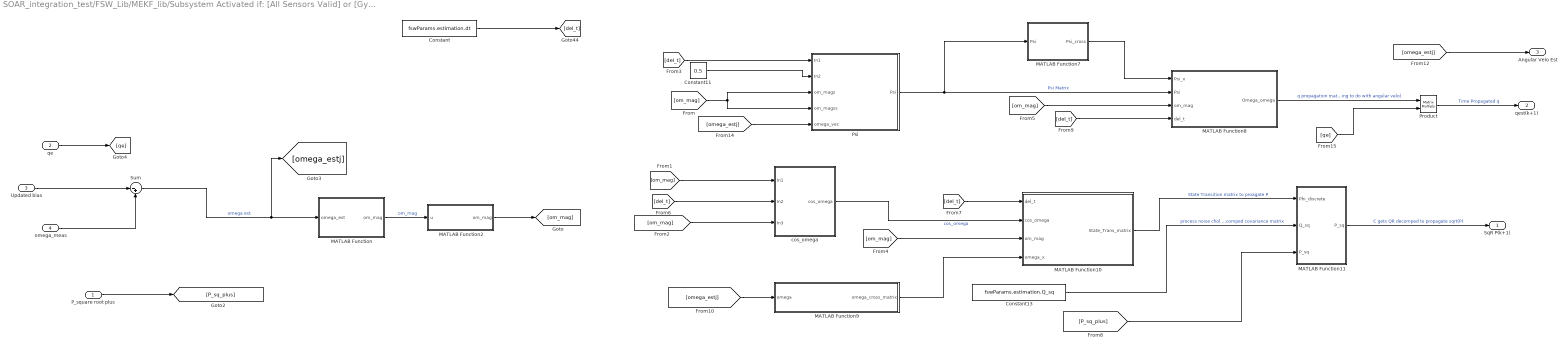
== system SOAR_integration_test/FSW_Lib/MEKF_lib/Subsystem Activated if: [All Sensors Valid] or [Gyro Bad and Sun//Mag sensors Valid]/TIME PROPAGATION of Q_EST, COVARIANCE ==
  P_square root plus : Inport
  qe : Inport  Port=2
  Updated bias : Inport  Port=3
  omega_meas : Inport  Port=4
  Constant : Constant  Value=fswParams.estimation.dt
  Constant11 : Constant  Value=0.5
  Constant13 : Constant  Value=fswParams.estimation.Q_sq  VectorParams1D=off
  MATLAB Function : MATLAB Function  TreatAsAtomicUnit=on
  MATLAB Function10 : MATLAB Function  TreatAsAtomicUnit=on
  MATLAB Function11 : MATLAB Function  TreatAsAtomicUnit=on
  MATLAB Function2 : MATLAB Function  TreatAsAtomicUnit=on
  MATLAB Function7 : MATLAB Function  TreatAsAtomicUnit=on
  MATLAB Function8 : MATLAB Function  TreatAsAtomicUnit=on
  MATLAB Function9 : MATLAB Function  TreatAsAtomicUnit=on
  Product : Product  Multiplication=Matrix(*)
  Psi : Subsystem
  Sum : Sum  Inputs=|-+
  cos_omega : Subsystem
  SqR P(k+1) : Outport
  qest(k+1) : Outport  Port=2
  Angular Velo Est : Outport  Port=3
  wires:
  MATLAB Function2/1(om_mag) -> [om_mag]
  [del_t] -> cos_omega/2(In2)
  Sum/1 -> MATLAB Function/1(omega_est), [omega_estj]  "omega est"
  [om_mag] -> Psi/4(om_magss), Psi/3(om_mags)
  [omega_estj] -> Psi/5(omega_vec)
  Constant11/1 -> Psi/2(In2)
  [del_t] -> Psi/1(In1)
  Psi/1(Psi) -> MATLAB Function7/1(Psi), MATLAB Function8/2(Psi)  "Psi Matrix"
  cos_omega/1(cos_omega) -> MATLAB Function10/2(cos_omega)  "cos_omega"
  [om_mag] -> cos_omega/3(In3)
  [om_mag] -> cos_omega/1(In1)
  [qe] -> Product/2
  [omega_estj] -> MATLAB Function9/1(omega)
  [om_mag] -> MATLAB Function8/3(om_mag)
  MATLAB Function/1(om_mag) -> MATLAB Function2/1(u)  "om_mag"
  Constant13/1 -> MATLAB Function11/2(Q_sq)  "process noise chol decomped covariance matrix"
  Product/1 -> qest(k+1)/1  "Time Propagated q"
  MATLAB Function10/1(State_Trans_matrix) -> MATLAB Function11/1(Phi_discrete)  "State Transition matrix to proagate P"
  MATLAB Function9/1(omega_cross_matrix) -> MATLAB Function10/4(omega_x)
  MATLAB Function8/1(Omega_omega) -> Product/1  "q propagation matrix (nothing to do with angular velo)"
  MATLAB Function11/1(P_sq) -> SqR P(k+1)/1  "C gets QR decomped to propagate sqrt(P)"
  MATLAB Function7/1(Psi_cross) -> MATLAB Function8/1(Psi_x)
  [del_t] -> MATLAB Function8/4(del_t)
  qe/1 -> [qe]
  Updated bias/1 -> Sum/1
  omega_meas/1 -> Sum/2
  P_square root plus/1 -> [P_sq_plus]
  [omega_estj] -> Angular Velo Est/1
  Constant/1 -> [del_t]
  [del_t] -> MATLAB Function10/1(del_t)
  [om_mag] -> MATLAB Function10/3(om_mag)
  [P_sq_plus] -> MATLAB Function11/3("P_sq ")

== system SOAR_integration_test/FSW_Lib/MEKF_lib/Subsystem Activated if: [Sun//Mag Sensor Invalid and Gyros are Valid] or [Gyro Invalid and Sun//Mag sensors Invalid]/Subsystem2 ==
  Square Root Covariane at next Time step becomes sqrt Pk minus : Inport
  Matrix Multiply : Product  Multiplication=Matrix(*)
  Transpose : Math  Operator=transpose  SaturateOnIntegerOverflow=on
  Out1 : Outport
  wires:
  Square Root Covariane at next Time step becomes sqrt Pk minus/1 -> Matrix Multiply/1, Transpose/1
  Transpose/1 -> Matrix Multiply/2
  Matrix Multiply/1 -> Out1/1

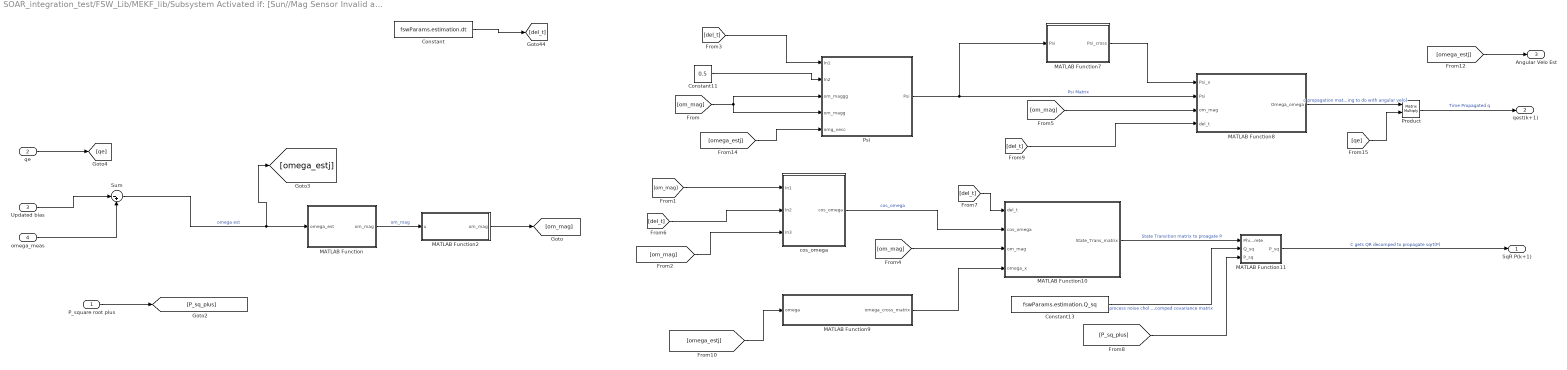
== system SOAR_integration_test/FSW_Lib/MEKF_lib/Subsystem Activated if: [Sun//Mag Sensor Invalid and Gyros are Valid] or [Gyro Invalid and Sun//Mag sensors Invalid]/TIME PROPAGATION of Q_EST, COVARIANCE ==
  P_square root plus : Inport
  qe : Inport  Port=2
  Updated bias : Inport  Port=3
  omega_meas : Inport  Port=4
  Constant : Constant  Value=fswParams.estimation.dt
  Constant11 : Constant  Value=0.5
  Constant13 : Constant  Value=fswParams.estimation.Q_sq  VectorParams1D=off
  MATLAB Function : MATLAB Function  TreatAsAtomicUnit=on
  MATLAB Function10 : MATLAB Function  TreatAsAtomicUnit=on
  MATLAB Function11 : MATLAB Function  TreatAsAtomicUnit=on
  MATLAB Function2 : MATLAB Function  TreatAsAtomicUnit=on
  MATLAB Function7 : MATLAB Function  TreatAsAtomicUnit=on
  MATLAB Function8 : MATLAB Function  TreatAsAtomicUnit=on
  MATLAB Function9 : MATLAB Function  TreatAsAtomicUnit=on
  Product : Product  Multiplication=Matrix(*)
  Psi : Subsystem
  Sum : Sum  Inputs=|-+
  cos_omega : Subsystem
  SqR P(k+1) : Outport
  qest(k+1) : Outport  Port=2
  Angular Velo Est : Outport  Port=3
  wires:
  [del_t] -> MATLAB Function8/4(del_t)
  MATLAB Function7/1(Psi_cross) -> MATLAB Function8/1(Psi_x)
  MATLAB Function11/1(P_sq) -> SqR P(k+1)/1  "C gets QR decomped to propagate sqrt(P)"
  MATLAB Function8/1(Omega_omega) -> Product/1  "q propagation matrix (nothing to do with angular velo)"
  MATLAB Function9/1(omega_cross_matrix) -> MATLAB Function10/4(omega_x)
  MATLAB Function10/1(State_Trans_matrix) -> MATLAB Function11/1(Phi_discrete)  "State Transition matrix to proagate P"
  Product/1 -> qest(k+1)/1  "Time Propagated q"
  Constant13/1 -> MATLAB Function11/2(Q_sq)  "process noise chol decomped covariance matrix"
  omega_meas/1 -> Sum/2
  Updated bias/1 -> Sum/1
  MATLAB Function/1(om_mag) -> MATLAB Function2/1(u)  "om_mag"
  [om_mag] -> MATLAB Function10/3(om_mag)
  [om_mag] -> MATLAB Function8/3(om_mag)
  [del_t] -> MATLAB Function10/1(del_t)
  P_square root plus/1 -> [P_sq_plus]
  [P_sq_plus] -> MATLAB Function11/3("P_sq ")
  [omega_estj] -> MATLAB Function9/1(omega)
  [omega_estj] -> Angular Velo Est/1
  qe/1 -> [qe]
  [qe] -> Product/2
  [om_mag] -> cos_omega/1(In1)
  [om_mag] -> cos_omega/3(In3)
  cos_omega/1(cos_omega) -> MATLAB Function10/2(cos_omega)  "cos_omega"
  Psi/1(Psi) -> MATLAB Function8/2(Psi), MATLAB Function7/1(Psi)  "Psi Matrix"
  [del_t] -> Psi/1(In1)
  Constant11/1 -> Psi/2(In2)
  [omega_estj] -> Psi/5(omg_vecc)
  [om_mag] -> Psi/3(om_maggg), Psi/4(om_magg)
  Sum/1 -> [omega_estj], MATLAB Function/1(omega_est)  "omega est"
  [del_t] -> cos_omega/2(In2)
  Constant/1 -> [del_t]
  MATLAB Function2/1(om_mag) -> [om_mag]

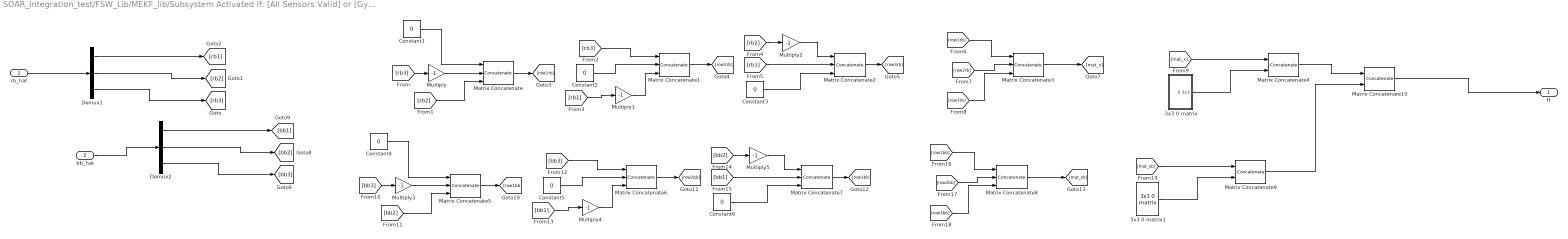
== system SOAR_integration_test/FSW_Lib/MEKF_lib/Subsystem Activated if: [All Sensors Valid] or [Gyro Bad and Sun//Mag sensors Valid]/Kalman Gain/Create H matrix ==
  rb_hat : Inport
  bb_hat : Inport  Port=2
  3x3 0 matrix : Subsystem
  3x3 0 matrix1 : MEKF_lib/MEKF_lib/Subsystem Activated if: [All Sensors Valid] or [Gyro Bad and Sun//Mag sensors Valid]/Kalman Gain/Create H matrix/3x3 0 matrix  SystemSampleTime=-1
  Constant{1..6} (6 alike) : Constant  Value=0
  Demux1 : Demux  Outputs=3
  Demux2 : Demux  Outputs=3
  Matrix Concatenate{,1..2,5..7} (6 alike) : Concatenate  NumInputs=3  Mode=Multidimensional array  ConcatenateDimension=2
  Matrix Concatenate10 : Concatenate  Mode=Multidimensional array
  Matrix Concatenate3 : Concatenate  NumInputs=3  Mode=Multidimensional array
  Matrix Concatenate4 : Concatenate  Mode=Multidimensional array  ConcatenateDimension=2
  Matrix Concatenate8 : Concatenate  NumInputs=3  Mode=Multidimensional array
  Matrix Concatenate9 : Concatenate  Mode=Multidimensional array  ConcatenateDimension=2
  Multiply{,1..5} (6 alike) : Gain  Gain=-1
  H : Outport
  wires:
  Matrix Concatenate10/1 -> H/1
  Matrix Concatenate4/1 -> Matrix Concatenate10/1
  [mat_xb] -> Matrix Concatenate9/1
  Matrix Concatenate9/1 -> Matrix Concatenate10/2
  3x3 0 matrix1/1 -> Matrix Concatenate9/2
  [row3bb] -> Matrix Concatenate8/3
  [row2bb] -> Matrix Concatenate8/2
  Matrix Concatenate8/1 -> [mat_xb]
  [row1bb] -> Matrix Concatenate8/1
  Matrix Concatenate6/1 -> [row2bb]
  [bb2] -> Multiply5/1
  [bb3] -> Matrix Concatenate6/1
  [bb3] -> Multiply3/1
  [bb2] -> Matrix Concatenate5/3
  Constant6/1 -> Matrix Concatenate7/3
  Matrix Concatenate7/1 -> [row3bb]
  [bb1] -> Multiply4/1
  Matrix Concatenate5/1 -> [row1bb]
  Multiply4/1 -> Matrix Concatenate6/3
  Constant5/1 -> Matrix Concatenate6/2
  Multiply3/1 -> Matrix Concatenate5/2
  Constant4/1 -> Matrix Concatenate5/1
  [bb1] -> Matrix Concatenate7/2
  Multiply5/1 -> Matrix Concatenate7/1
  Demux2/2 -> [bb2]
  Demux2/1 -> [bb1]
  bb_hat/1 -> Demux2/1
  Demux2/3 -> [bb3]
  rb_hat/1 -> Demux1/1
  Demux1/3 -> [rb3]
  [rb1] -> Matrix Concatenate2/2
  Constant2/1 -> Matrix Concatenate1/2
  Matrix Concatenate3/1 -> [mat_x]
  Demux1/1 -> [rb1]
  [row1rb] -> Matrix Concatenate3/1
  Constant1/1 -> Matrix Concatenate/1
  [row2rb] -> Matrix Concatenate3/2
  [rb3] -> Matrix Concatenate1/1
  [rb2] -> Matrix Concatenate/3
  [rb2] -> Multiply2/1
  3x3 0 matrix/1(0 3x3) -> Matrix Concatenate4/2
  Constant3/1 -> Matrix Concatenate2/3
  Multiply1/1 -> Matrix Concatenate1/3
  [rb3] -> Multiply/1
  [rb1] -> Multiply1/1
  Matrix Concatenate2/1 -> [row3rb]
  Matrix Concatenate/1 -> [row1rb]
  [row3rb] -> Matrix Concatenate3/3
  Multiply2/1 -> Matrix Concatenate2/1
  Demux1/2 -> [rb2]
  [mat_x] -> Matrix Concatenate4/1
  Multiply/1 -> Matrix Concatenate/2
  Matrix Concatenate1/1 -> [row2rb]

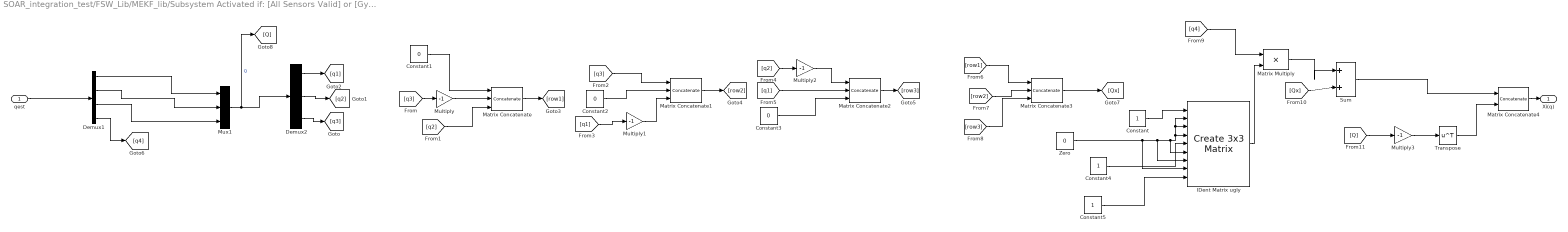
== system SOAR_integration_test/FSW_Lib/MEKF_lib/Subsystem Activated if: [All Sensors Valid] or [Gyro Bad and Sun//Mag sensors Valid]/Kalman Gain/Makes Xi(q) Matrix ==
  qest : Inport
  Constant : Constant
  Constant1 : Constant  Value=0
  Constant2 : Constant  Value=0
  Constant3 : Constant  Value=0
  Constant4 : Constant
  Constant5 : Constant
  Demux1 : Demux
  Demux2 : Demux  Outputs=3
  IDent Matrix ugly : sharedutil/Create 3x3 Matrix  aMode=aMode
  Matrix Concatenate : Concatenate  NumInputs=3  Mode=Multidimensional array  ConcatenateDimension=2
  Matrix Concatenate1 : Concatenate  NumInputs=3  Mode=Multidimensional array  ConcatenateDimension=2
  Matrix Concatenate2 : Concatenate  NumInputs=3  Mode=Multidimensional array  ConcatenateDimension=2
  Matrix Concatenate3 : Concatenate  NumInputs=3  Mode=Multidimensional array
  Matrix Concatenate4 : Concatenate  Mode=Multidimensional array
  Matrix Multiply : Product  Inputs=**
  Multiply{,1..3} (4 alike) : Gain  Gain=-1
  Mux1 : Mux  Inputs=3
  Sum : Sum  Inputs=|++
  Transpose : Math  Operator=transpose  SaturateOnIntegerOverflow=on
  Zero : Constant  Value=0  OutDataTypeStr=Inherit: Inherit via back propagation
  Xi(q) : Outport
  wires:
  Zero/1 -> IDent Matrix ugly/2, IDent Matrix ugly/3, IDent Matrix ugly/4, IDent Matrix ugly/6, IDent Matrix ugly/7, IDent Matrix ugly/8
  Constant4/1 -> IDent Matrix ugly/5
  Constant5/1 -> IDent Matrix ugly/9
  Constant/1 -> IDent Matrix ugly/1
  Matrix Concatenate4/1 -> Xi(q)/1
  Multiply1/1 -> Matrix Concatenate1/3
  [q1] -> Multiply1/1
  Constant3/1 -> Matrix Concatenate2/3
  Demux2/3 -> [q3]
  Matrix Concatenate/1 -> [row1]
  [q3] -> Multiply/1
  IDent Matrix ugly/1 -> Matrix Multiply/2
  Transpose/1 -> Matrix Concatenate4/2
  Demux2/1 -> [q1]
  [Q] -> Multiply3/1
  [row1] -> Matrix Concatenate3/1
  Multiply/1 -> Matrix Concatenate/2
  [Qx] -> Sum/2
  Matrix Concatenate2/1 -> [row3]
  Demux1/3 -> Mux1/3
  Demux1/1 -> Mux1/1
  [row2] -> Matrix Concatenate3/2
  Demux1/4 -> [q4]
  [q2] -> Multiply2/1
  Sum/1 -> Matrix Concatenate4/1
  Demux2/2 -> [q2]
  [q3] -> Matrix Concatenate1/1
  [q4] -> Matrix Multiply/1
  Multiply3/1 -> Transpose/1
  qest/1 -> Demux1/1
  [row3] -> Matrix Concatenate3/3
  Demux1/2 -> Mux1/2
  Constant2/1 -> Matrix Concatenate1/2
  Mux1/1 -> [Q], Demux2/1  "Q"
  [q2] -> Matrix Concatenate/3
  Matrix Concatenate3/1 -> [Qx]
  Constant1/1 -> Matrix Concatenate/1
  Matrix Concatenate1/1 -> [row2]
  Matrix Multiply/1 -> Sum/1
  [q1] -> Matrix Concatenate2/2
  Multiply2/1 -> Matrix Concatenate2/1

== system SOAR_integration_test/FSW_Lib/MEKF_lib/Subsystem Activated if: [All Sensors Valid] or [Gyro Bad and Sun//Mag sensors Valid]/MEASUREMENT UPDATE TO q AND COVARIANCE2/Normalize_q ==
  note: Rearrange_Quat_back
  note: Rearrange_Quat
  Estimated Quaternion : Inport
  Demux : Demux
  Demux1 : Demux
  Mux : Mux
  Mux1 : Mux
  Quaternion Normalize : sharedutil/Quaternion Normalize  aMode=aMode
      settings: SourceProductName=Aerospace Blockset  SourceProductBaseCode=AE
  q_normalized : Outport
  wires:
  Estimated Quaternion/1 -> Demux1/1
  Quaternion Normalize/1 -> Demux/1  "Measurement updated q estimate"
  Demux/1 -> Mux/4
  Demux1/2 -> Mux1/3
  Demux1/1 -> Mux1/2
  Mux/1 -> q_normalized/1
  Demux1/3 -> Mux1/4
  Demux/2 -> Mux/1
  Demux/3 -> Mux/2
  Demux/4 -> Mux/3
  Demux1/4 -> Mux1/1
  Mux1/1 -> Quaternion Normalize/1

== system SOAR_integration_test/FSW_Lib/MEKF_lib/Subsystem Activated if: [All Sensors Valid] or [Gyro Bad and Sun//Mag sensors Valid]/TIME PROPAGATION of Q_EST, COVARIANCE/Psi ==
  In1 : Inport
  In2 : Inport  Port=2
  om_mags : Inport  Port=3
  om_magss : Inport  Port=4
  omega_vec : Inport  Port=5
  Divide : Product  Inputs=***
  Divide1 : Product  Inputs=**/
  Sin : Trigonometry
  Psi : Outport
  wires:
  om_magss/1 -> Divide1/3
  omega_vec/1 -> Divide1/2
  In2/1 -> Divide/2
  Sin/1 -> Divide1/1  "sin(om_mag*0.5*del_t)"
  om_mags/1 -> Divide/3
  Divide1/1 -> Psi/1  "Psi"
  Divide/1 -> Sin/1  "om_mag times0.5*del_t"
  In1/1 -> Divide/1

== system SOAR_integration_test/FSW_Lib/MEKF_lib/Subsystem Activated if: [All Sensors Valid] or [Gyro Bad and Sun//Mag sensors Valid]/TIME PROPAGATION of Q_EST, COVARIANCE/cos_omega ==
  In1 : Inport
  In2 : Inport  Port=2
  In3 : Inport  Port=3
  Constant12 : Constant
  Cos : Trigonometry  Operator=cos
  Divide2 : Product  Inputs=**
  Divide3 : Product  Inputs=*/
  Square : Math  Operator=square  SaturateOnIntegerOverflow=on
  Sum3 : Sum  Inputs=|+-
  cos_omega : Outport
  wires:
  Sum3/1 -> Divide3/1  "(1-cos(om_mag*del_t))"
  In2/1 -> Divide2/2
  Cos/1 -> Sum3/2
  In1/1 -> Divide2/1
  Square/1 -> Divide3/2  "omega mag squared"
  Constant12/1 -> Sum3/1
  Divide3/1 -> cos_omega/1  "cos_omega"
  In3/1 -> Square/1
  Divide2/1 -> Cos/1

== system SOAR_integration_test/FSW_Lib/MEKF_lib/Subsystem Activated if: [Sun//Mag Sensor Invalid and Gyros are Valid] or [Gyro Invalid and Sun//Mag sensors Invalid]/TIME PROPAGATION of Q_EST, COVARIANCE/Psi ==
  In1 : Inport
  In2 : Inport  Port=2
  om_maggg : Inport  Port=3
  om_magg : Inport  Port=4
  omg_vecc : Inport  Port=5
  Divide : Product  Inputs=***
  Divide1 : Product  Inputs=**/
  Sin : Trigonometry
  Psi : Outport
  wires:
  In1/1 -> Divide/1
  Divide/1 -> Sin/1  "om_mag times0.5*del_t"
  om_magg/1 -> Divide1/3
  omg_vecc/1 -> Divide1/2
  Divide1/1 -> Psi/1  "Psi"
  om_maggg/1 -> Divide/3
  Sin/1 -> Divide1/1  "sin(om_mag*0.5*del_t)"
  In2/1 -> Divide/2

== system SOAR_integration_test/FSW_Lib/MEKF_lib/Subsystem Activated if: [Sun//Mag Sensor Invalid and Gyros are Valid] or [Gyro Invalid and Sun//Mag sensors Invalid]/TIME PROPAGATION of Q_EST, COVARIANCE/cos_omega ==
  In1 : Inport
  In2 : Inport  Port=2
  In3 : Inport  Port=3
  Constant12 : Constant
  Cos : Trigonometry  Operator=cos
  Divide2 : Product  Inputs=**
  Divide3 : Product  Inputs=*/
  Square : Math  Operator=square  SaturateOnIntegerOverflow=on
  Sum3 : Sum  Inputs=|+-
  cos_omega : Outport
  wires:
  Divide2/1 -> Cos/1
  In3/1 -> Square/1
  Divide3/1 -> cos_omega/1  "cos_omega"
  Constant12/1 -> Sum3/1
  Square/1 -> Divide3/2  "omega mag squared"
  In1/1 -> Divide2/1
  Cos/1 -> Sum3/2
  In2/1 -> Divide2/2
  Sum3/1 -> Divide3/1  "(1-cos(om_mag*del_t))"

== system SOAR_integration_test/FSW_Lib/MEKF_lib/Subsystem Activated if: [All Sensors Valid] or [Gyro Bad and Sun//Mag sensors Valid]/Kalman Gain/Create H matrix/3x3 0 matrix ==
  Create 3x3 Matrix : sharedutil/Create 3x3 Matrix  aMode=aMode
  Zero : Constant  Value=0  OutDataTypeStr=Inherit: Inherit via back propagation
  0 3x3 : Outport
  wires:
  Create 3x3 Matrix/1 -> 0 3x3/1
  Zero/1 -> Create 3x3 Matrix/4, Create 3x3 Matrix/3, Create 3x3 Matrix/2, Create 3x3 Matrix/5, Create 3x3 Matrix/1, Create 3x3 Matrix/6, Create 3x3 Matrix/7, Create 3x3 Matrix/8, Create 3x3 Matrix/9

== matlab function SOAR_integration_test/FSW_Lib/MEKF_lib/Subsystem Activated if: [Sun//Mag Sensor Invalid and Gyros are Valid] or [Gyro Invalid and Sun//Mag sensors Invalid]/TIME PROPAGATION of Q_EST, COVARIANCE/MATLAB Function ==
  data: omega_est input; om_mag output
function om_mag = om2_norm(omega_est)

om_mag = norm(omega_est);

== matlab function SOAR_integration_test/FSW_Lib/MEKF_lib/Subsystem Activated if: [Sun//Mag Sensor Invalid and Gyros are Valid] or [Gyro Invalid and Sun//Mag sensors Invalid]/TIME PROPAGATION of Q_EST, COVARIANCE/MATLAB Function10 ==
  data: del_t input; cos_omega input; om_mag input; omega_x input; State_Trans_matrix output
function State_Trans_matrix = Phi_disc(del_t,cos_omega,om_mag,omega_x)
%#codegen

State_Trans_matrix = [(eye(3)-omega_x*sin(om_mag*del_t)/om_mag + (omega_x^2)*cos_omega),omega_x*cos_omega-eye(3)*del_t-omega_x^2*(om_mag*del_t-sin(om_mag*del_t))/om_mag^3;
            zeros(3,3),eye(3)];

== matlab function SOAR_integration_test/FSW_Lib/MEKF_lib/Subsystem Activated if: [All Sensors Valid] or [Gyro Bad and Sun//Mag sensors Valid]/Kalman Gain/MATLAB Function2 ==
  data: P_sq output; R_sq input; K output; P_sq input; H input
function [P_sq,K] = fcnAQR(R_sq,P_sq,H)
%#codegen
[nr,mr] = size(R_sq);
[np,mp] = size(P_sq);
A_QR = [R_sq',zeros(nr,np);(P_sq')*H', P_sq'];

[TA,UA] = qr(A_QR);
        P_sq = UA(7:12,7:12)'; %Updated P_sq
        W = UA(1:6,7:12)';
%        
        sq_Bk = UA(1:6,1:6)';
        
       
         K = W*inv(sq_Bk);

== matlab function SOAR_integration_test/FSW_Lib/MEKF_lib/Subsystem Activated if: [Sun//Mag Sensor Invalid and Gyros are Valid] or [Gyro Invalid and Sun//Mag sensors Invalid]/TIME PROPAGATION of Q_EST, COVARIANCE/MATLAB Function11 ==
  data: Phi_discrete input; P_sq output; Q_sq input; P_sq input
function P_sq  = Cqr(Phi_discrete,Q_sq,P_sq)
%#codegen

C = [P_sq'*Phi_discrete';Q_sq'];
          [Tc,Uc] = qr(C);
%           Uc = full(Uc);
          sq_P_kp1 = Uc(1:6,1:6)';
%           P = sq_P_kp1'*sq_P_kp1;
          P_sq = sq_P_kp1;

== matlab function SOAR_integration_test/FSW_Lib/MEKF_lib/Subsystem Activated if: [Sun//Mag Sensor Invalid and Gyros are Valid] or [Gyro Invalid and Sun//Mag sensors Invalid]/TIME PROPAGATION of Q_EST, COVARIANCE/MATLAB Function2 ==
  data: u input; om_mag output
function om_mag = norm_check1(u)
%#codegen
if u == 0
    om_mag = 10^-10;
else
    om_mag = u;
end

end

== matlab function SOAR_integration_test/FSW_Lib/MEKF_lib/Subsystem Activated if: [Sun//Mag Sensor Invalid and Gyros are Valid] or [Gyro Invalid and Sun//Mag sensors Invalid]/TIME PROPAGATION of Q_EST, COVARIANCE/MATLAB Function7 ==
  data: Psi input; Psi_cross output
function Psi_cross = Psi_cross_matrix(Psi)
%#codegen

Psi_cross = [0 -Psi(3) Psi(2);Psi(3) 0 -Psi(1);-Psi(2) Psi(1) 0];

== matlab function SOAR_integration_test/FSW_Lib/MEKF_lib/Subsystem Activated if: [Sun//Mag Sensor Invalid and Gyros are Valid] or [Gyro Invalid and Sun//Mag sensors Invalid]/TIME PROPAGATION of Q_EST, COVARIANCE/MATLAB Function8 ==
  data: Psi_x input; Psi input; om_mag input; del_t input; Omega_omega output
function Omega_omega = omega_omega_matrix(Psi_x,Psi,om_mag,del_t)
%#codegen

 Omega_omega = [(cos(0.5*om_mag*del_t)*eye(3) - Psi_x), Psi; -Psi', cos(0.5*om_mag*del_t)];

== matlab function SOAR_integration_test/FSW_Lib/MEKF_lib/Subsystem Activated if: [All Sensors Valid] or [Gyro Bad and Sun//Mag sensors Valid]/TIME PROPAGATION of Q_EST, COVARIANCE/MATLAB Function7 ==
  data: Psi input; Psi_cross output
function Psi_cross = Psi_cross_matrix(Psi)
%#codegen

Psi_cross = [0 -Psi(3) Psi(2);Psi(3) 0 -Psi(1);-Psi(2) Psi(1) 0];

== matlab function SOAR_integration_test/FSW_Lib/MEKF_lib/Subsystem Activated if: [All Sensors Valid] or [Gyro Bad and Sun//Mag sensors Valid]/TIME PROPAGATION of Q_EST, COVARIANCE/MATLAB Function8 ==
  data: Psi_x input; Psi input; om_mag input; del_t input; Omega_omega output
function Omega_omega = omega_omega_matrix(Psi_x,Psi,om_mag,del_t)
%#codegen

 Omega_omega = [(cos(0.5*om_mag*del_t)*eye(3) - Psi_x), Psi; -Psi', cos(0.5*om_mag*del_t)];

== matlab function SOAR_integration_test/FSW_Lib/MEKF_lib/Subsystem Activated if: [All Sensors Valid] or [Gyro Bad and Sun//Mag sensors Valid]/TIME PROPAGATION of Q_EST, COVARIANCE/MATLAB Function9 ==
  data: omega input; omega_cross_matrix output
function omega_cross_matrix = makes_omega_cross_matrix(omega)

omega_cross_matrix = [0 -omega(3) omega(2);omega(3) 0 -omega(1);-omega(2) omega(1) 0];

== matlab function SOAR_integration_test/FSW_Lib/MEKF_lib/Subsystem Activated if: [All Sensors Valid] or [Gyro Bad and Sun//Mag sensors Valid]/TIME PROPAGATION of Q_EST, COVARIANCE/MATLAB Function10 ==
  data: del_t input; cos_omega input; om_mag input; omega_x input; State_Trans_matrix output
function State_Trans_matrix = Phi_disc(del_t,cos_omega,om_mag,omega_x)
%#codegen

State_Trans_matrix = [(eye(3)-omega_x*sin(om_mag*del_t)/om_mag + (omega_x^2)*cos_omega),omega_x*cos_omega-eye(3)*del_t-omega_x^2*(om_mag*del_t-sin(om_mag*del_t))/om_mag^3;
            zeros(3,3),eye(3)];
